simulink model "inv2_2x3_inv3_3x4_inv4"  (R2017b)
settings: Solver=FixedStepDiscrete  StartTime=0.0  StopTime=19.8  FixedStep=0.200000  RelTol=1e-3
model workspace (MAT data in the model file):
  already_pp = 0
  input_struct.time = [0; 0.2; 0.4; 0.6; 0.8; 1; 1.2; 1.4; 1.6; 1.8; 2; 2.2; 2.4; 2.6; 2.8; 3; 3.2; 3.4; 3.6; 3.8; 4; 4.2; 4.4; 4.6; 4.8; 5; 5.2; 5.4; 5.6; 5.8; 6; 6.2; 6.4; 6.6; 6.8; 7; 7.2; 7.4; 7.6; 7.8; 8; 8.2; 8.4; 8.6; 8.8; 9; 9.2; 9.4; 9.6; 9.8; 10; 10.2; 10.4; 10.6; 10.8; 11; 11.2; 11.4; 11.6; 11.8; 12; 12.2; 12.4; 12.6; 12.8; 13; 13.2; 13.4; 13.6; 13.8; 14; 14.2; 14.4; 14.6; 14.8; 15; 15.2; 15.4; 15.6; 15.8; 16; 16.2; 16.4; 16.6; 16.8; 17; 17.2; 17.4; 17.6; 17.8; 18; 18.2; 18.4; 18.6; 18.8; 19; 19.2; 19.4; 19.6; 19.8]
  input_struct.signals(1).name = 'A'
  input_struct.signals(1).values = [-67.7798567966 -284.294456785 80.1278430703 39.1506354271 -80.6931523013 -47.1247806845 -22.6798367824 -111.336734366 -164.602985191 -230.437869558 -219.620336593 267.914066196 ... (400 elements, 2x2x100)]
  input_struct.signals(1).dimensions = [2 2]
  input_struct.signals(2).name = 'B'
  input_struct.signals(2).values = [-259.532331725 92.0939128985 -153.42865549 154.750939948 -120.591477651 -48.7109432253 -266.500683747 -281.486208073 -188.051769572 -137.456610468 -260.25402492 -99.9037845224 ... (600 elements, 2x3x100)]
  input_struct.signals(2).dimensions = [2 3]
  input_struct.signals(3).name = 'B1'
  input_struct.signals(3).values = [145.896759474 -213.413285754 -259.040943569 19.2819230591 146.373170049 201.440171451 132.3977907 232.573567412 -202.287973125 -179.256093004 229.176919402 -22.8246387267 ... (900 elements, 3x3x100)]
  input_struct.signals(3).dimensions = [3 3]
  input_struct.signals(4).name = 'B2'
  input_struct.signals(4).values = [125.478179701 -221.822687201 14.3983643337 -272.465931463 -239.216587216 -18.6389460851 126.387817451 60.8078445021 -177.049814306 71.2719160314 119.490067991 -111.102797989 ... (1200 elements, 3x4x100)]
  input_struct.signals(4).dimensions = [3 4]
  input_struct.signals(5).name = 'B3'
  input_struct.signals(5).values = [-92.1749382408 91.3231619298 -10.9455289927 -70.4438170619 -103.868495876 -238.17604952 -77.7525724158 -73.5350762415 -10.9210075339 177.371737726 114.836217702 209.874059192 ... (1600 elements, 4x4x100)]
  input_struct.signals(5).dimensions = [4 4]
settings Model: Creator=ktrinh  LastModifiedBy=hbourbou
settings DataIOCC: ExternalInput=input_struct  LoadExternalInput=on  SaveFormat=Structure  SaveState=on
settings OptimizationCC: LifeSpan=inf
settings DebuggingCC: AlgebraicLoopMsg=error  ArtificialAlgebraicLoopMsg=error  SFExecutionAtInitializationDiag=none
settings HardwareCC: ProdBitPerSizeT=32  ProdBitPerPtrDiffT=32  ProdWordSize=32  ProdHWDeviceType=Specified
settings CodeAppCC: StateflowObjectComments=on
settings GRTTargetCC: ExtMode=on

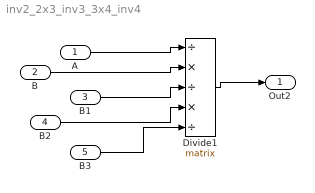
== system inv2_2x3_inv3_3x4_inv4 ==
  A : Inport  OutDataTypeStr=double  PortDimensions=[2 2]
  B : Inport  Port=2  OutDataTypeStr=double  PortDimensions=[2 3]
  B1 : Inport  Port=3  OutDataTypeStr=double  PortDimensions=[3 3]
  B2 : Inport  Port=4  OutDataTypeStr=double  PortDimensions=[3 4]
  B3 : Inport  Port=5  OutDataTypeStr=double  PortDimensions=[4 4]
  Divide1 : Product  Inputs=/*/*/  Multiplication=Matrix(*)
  Out2 : Outport
  wires:
  A/1 -> Divide1/1
  Divide1/1 -> Out2/1
  B/1 -> Divide1/2
  B1/1 -> Divide1/3
  B2/1 -> Divide1/4
  B3/1 -> Divide1/5
